simulink model "MassSpringDamper"  (R2023b)
settings: Solver=VariableStepAuto  StartTime=0.0  StopTime=30  MaxStep=0.001  RelTol=1e-3
settings Model: Creator=Lakshmi  LastModifiedBy=Lakshmi

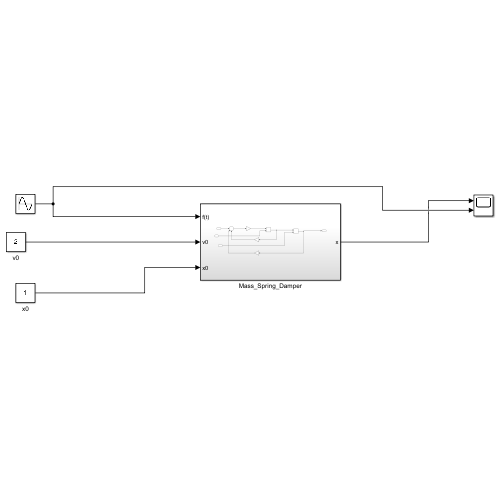
[thumbnail: Simulink's stored preview of the top-level diagram]
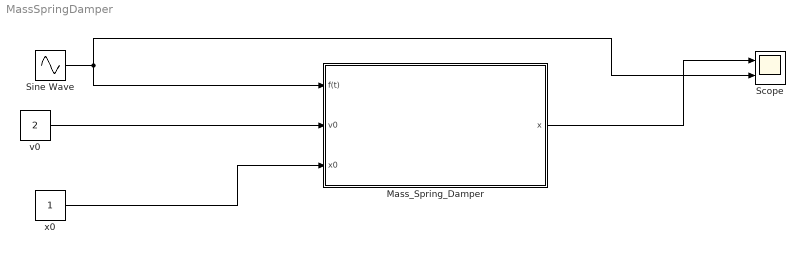
== system MassSpringDamper ==
  Mass_Spring_Damper : Subsystem
  Scope : Scope  NumInputPorts=2
  Sine Wave : Sin  Amplitude=2  Frequency=2  SampleTime=0
  v0 : Constant  Value=2
  x0 : Constant
  wires:
  Sine Wave/1 -> Mass_Spring_Damper/1(f(t)), Scope/2
  v0/1 -> Mass_Spring_Damper/2(v0)
  x0/1 -> Mass_Spring_Damper/3(x0)
  Mass_Spring_Damper/1(x) -> Scope/1

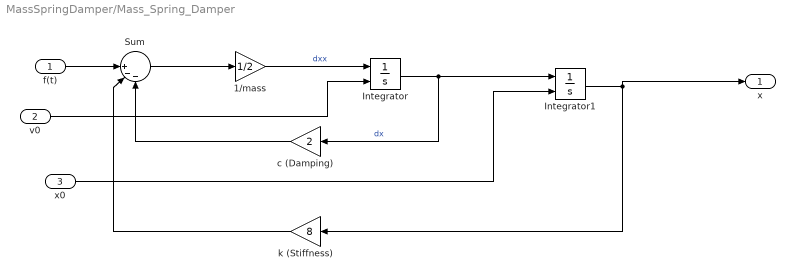
== system MassSpringDamper/Mass_Spring_Damper ==
  f(t) : Inport
  v0 : Inport  Port=2
  x0 : Inport  Port=3
  1/mass : Gain  Gain=1/2
  Integrator : Integrator  InitialConditionSource=external  InitialCondition=2
  Integrator1 : Integrator  InitialConditionSource=external  InitialCondition=1
  Sum : Sum  Inputs=||+--
  c (Damping) : Gain  Gain=2
  k (Stiffness) : Gain  Gain=8
  x : Outport
  wires:
  Integrator/1 -> Integrator1/1, c (Damping)/1  "dx"
  c (Damping)/1 -> Sum/3
  v0/1 -> Integrator/2
  Integrator1/1 -> x/1, k (Stiffness)/1
  1/mass/1 -> Integrator/1  "dxx"
  Sum/1 -> 1/mass/1
  k (Stiffness)/1 -> Sum/2
  x0/1 -> Integrator1/2
  f(t)/1 -> Sum/1
